simulink subsystem "InversePendulum"  (R2023a)
settings: Solver=VariableStepAuto  StartTime=0.0  StopTime=10.0  RelTol=1e-3
values from neighbouring files (symbols this model uses):
  g = 9.8    [constants.m]
  L = 350 * 10^-6    (= 0.00035)    [constants.m]
  m = .1    (= 0.1)    [constants.m]
  M = .2    (= 0.2)    [constants.m]
  ts = 3/7    (= 0.428571428571)    [constants.m]
settings Model: Creator=ycheb  LastModifiedBy=Edgar

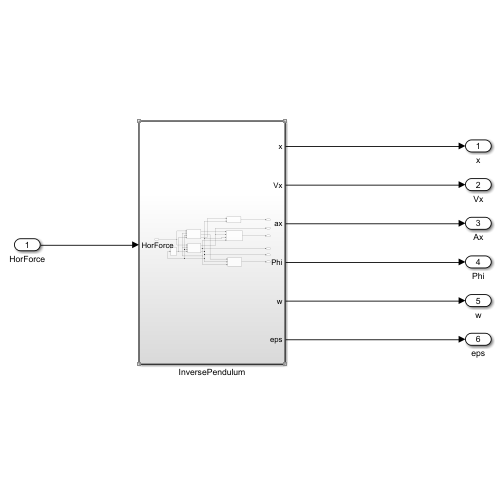
[thumbnail: Simulink's stored preview of the top-level diagram]
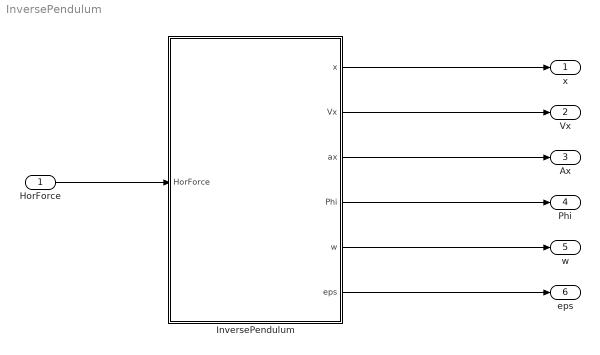
== system InversePendulum ==
  HorForce : Inport
  InversePendulum : Subsystem
  x : Outport
  Vx : Outport  Port=2
  Ax : Outport  Port=3
  Phi : Outport  Port=4
  w : Outport  Port=5
  eps : Outport  Port=6
  wires:
  InversePendulum/5(w) -> w/1
  InversePendulum/4(Phi) -> Phi/1
  InversePendulum/6(eps) -> eps/1
  InversePendulum/2(Vx) -> Vx/1
  HorForce/1 -> InversePendulum/1(HorForce)
  InversePendulum/3(ax) -> Ax/1
  InversePendulum/1(x) -> x/1

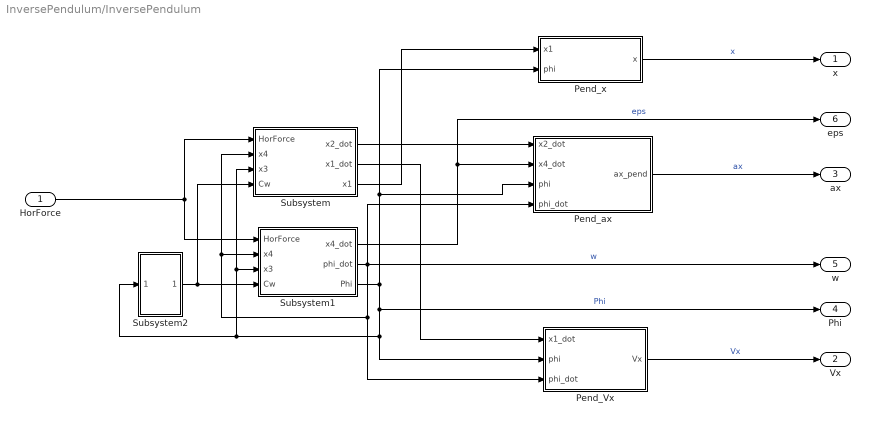
== system InversePendulum/InversePendulum ==
  HorForce : Inport
  Pend_Vx : Subsystem
  Pend_ax : Subsystem
  Pend_x : Subsystem
  Subsystem : Subsystem
  Subsystem1 : Subsystem
  Subsystem2 : Subsystem
  x : Outport
  Vx : Outport  Port=2
  ax : Outport  Port=3
  Phi : Outport  Port=4
  w : Outport  Port=5
  eps : Outport  Port=6
  wires:
  Subsystem1/2(phi_dot) -> w/1, Pend_ax/4(phi_dot), Pend_Vx/3(phi_dot), Subsystem/2(x4), Subsystem1/2(x4)  "w"
  Subsystem2/1(Cw) -> Subsystem/4(Cw), Subsystem1/4(Cw)
  HorForce/1 -> Subsystem1/1(HorForce), Subsystem/1(HorForce)
  Subsystem1/3(Phi) -> Phi/1, Pend_Vx/2(phi), Subsystem/3(x3), Subsystem1/3(x3), Subsystem2/1(Phi), Pend_x/2(phi), Pend_ax/3(phi)  "Phi"
  Pend_Vx/1(Vx) -> Vx/1  "Vx"
  Pend_ax/1(ax_pend) -> ax/1  "ax"
  Subsystem1/1(x4_dot) -> eps/1, Pend_ax/2(x4_dot)  "eps"
  Subsystem/1(x2_dot) -> Pend_ax/1(x2_dot)
  Subsystem/3(x1) -> Pend_x/1(x1)
  Subsystem/2(x1_dot) -> Pend_Vx/1(x1_dot)
  Pend_x/1(x) -> x/1  "x"

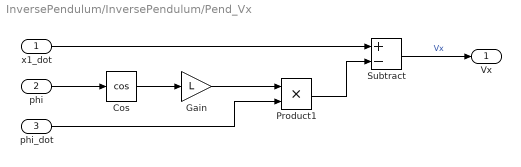
== system InversePendulum/InversePendulum/Pend_Vx ==
  x1_dot : Inport
  phi : Inport  Port=2
  phi_dot : Inport  Port=3
  Cos : Trigonometry  Operator=cos
  Gain : Gain  Gain=L
  Product1 : Product
  Subtract : Sum  Inputs=+-
  Vx : Outport
  wires:
  phi/1 -> Cos/1
  Subtract/1 -> Vx/1  "Vx"
  x1_dot/1 -> Subtract/1
  phi_dot/1 -> Product1/2
  Product1/1 -> Subtract/2
  Cos/1 -> Gain/1
  Gain/1 -> Product1/1

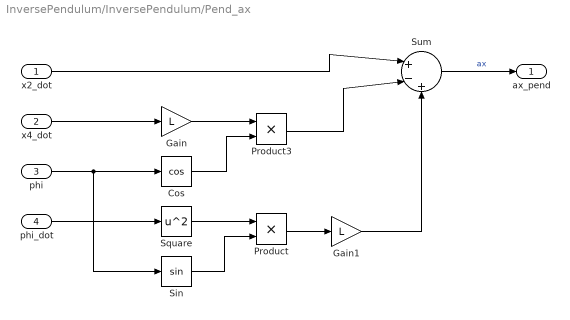
== system InversePendulum/InversePendulum/Pend_ax ==
  x2_dot : Inport
  x4_dot : Inport  Port=2
  phi : Inport  Port=3
  phi_dot : Inport  Port=4
  Cos : Trigonometry  Operator=cos
  Gain : Gain  Gain=L
  Gain1 : Gain  Gain=L
  Product : Product
  Product3 : Product
  Sin : Trigonometry
  Square : Math  Operator=square
  Sum : Sum  Inputs=|+-+
  ax_pend : Outport
  wires:
  x2_dot/1 -> Sum/1
  Sum/1 -> ax_pend/1  "ax"
  Gain/1 -> Product3/1
  Product3/1 -> Sum/2
  phi/1 -> Sin/1, Cos/1
  Cos/1 -> Product3/2
  x4_dot/1 -> Gain/1
  phi_dot/1 -> Square/1
  Square/1 -> Product/1
  Sin/1 -> Product/2
  Product/1 -> Gain1/1
  Gain1/1 -> Sum/3

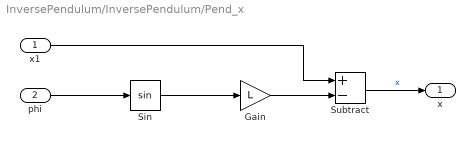
== system InversePendulum/InversePendulum/Pend_x ==
  x1 : Inport
  phi : Inport  Port=2
  Gain : Gain  Gain=L
  Sin : Trigonometry
  Subtract : Sum  Inputs=+-
  x : Outport
  wires:
  Sin/1 -> Gain/1
  Gain/1 -> Subtract/2
  Subtract/1 -> x/1  "x"
  x1/1 -> Subtract/1
  phi/1 -> Sin/1

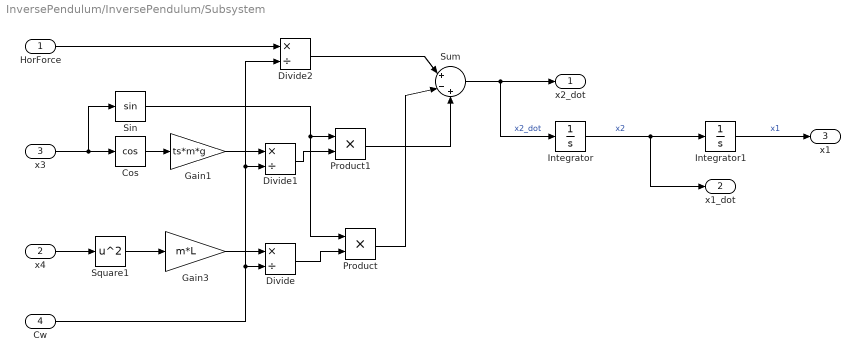
== system InversePendulum/InversePendulum/Subsystem ==
  HorForce : Inport
  x4 : Inport  Port=2
  x3 : Inport  Port=3
  Cw : Inport  Port=4
  Cos : Trigonometry  Operator=cos
  Divide : Product  Inputs=*/
  Divide1 : Product  Inputs=*/
  Divide2 : Product  Inputs=*/
  Gain1 : Gain  Gain=ts*m*g
  Gain3 : Gain  Gain=m*L
  Integrator : Integrator
  Integrator1 : Integrator
  Product : Product
  Product1 : Product
  Sin : Trigonometry
  Square1 : Math  Operator=square
  Sum : Sum  Inputs=|+-+
  x2_dot : Outport
  x1_dot : Outport  Port=2
  x1 : Outport  Port=3
  wires:
  Sum/1 -> Integrator/1, x2_dot/1  "x2_dot"
  Square1/1 -> Gain3/1
  Product/1 -> Sum/2
  x3/1 -> Sin/1, Cos/1
  x4/1 -> Square1/1
  Integrator/1 -> x1_dot/1, Integrator1/1  "x2"
  Integrator1/1 -> x1/1  "x1"
  Cos/1 -> Gain1/1
  Sin/1 -> Product/1, Product1/1
  Product1/1 -> Sum/3
  Gain3/1 -> Divide/1
  Cw/1 -> Divide/2, Divide2/2, Divide1/2
  Divide/1 -> Product/2
  Gain1/1 -> Divide1/1
  Divide1/1 -> Product1/2
  HorForce/1 -> Divide2/1
  Divide2/1 -> Sum/1

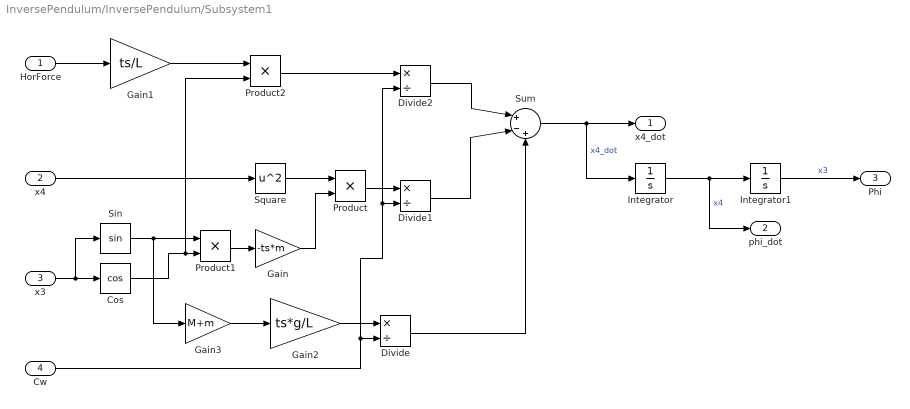
== system InversePendulum/InversePendulum/Subsystem1 ==
  HorForce : Inport
  x4 : Inport  Port=2
  x3 : Inport  Port=3
  Cw : Inport  Port=4
  Cos : Trigonometry  Operator=cos
  Divide : Product  Inputs=*/
  Divide1 : Product  Inputs=*/
  Divide2 : Product  Inputs=*/
  Gain : Gain  Gain=-ts*m
  Gain1 : Gain  Gain=ts/L
  Gain2 : Gain  Gain=ts*g/L
  Gain3 : Gain  Gain=M+m
  Integrator : Integrator
  Integrator1 : Integrator  InitialCondition=5*pi/180
  Product : Product
  Product1 : Product
  Product2 : Product
  Sin : Trigonometry
  Square : Math  Operator=square
  Sum : Sum  Inputs=|+-+
  x4_dot : Outport
  phi_dot : Outport  Port=2
  Phi : Outport  Port=3
  wires:
  Gain/1 -> Product/2
  x3/1 -> Cos/1, Sin/1
  Square/1 -> Product/1
  Gain3/1 -> Gain2/1
  Sum/1 -> Integrator/1, x4_dot/1  "x4_dot"
  HorForce/1 -> Gain1/1
  x4/1 -> Square/1
  Integrator/1 -> Integrator1/1, phi_dot/1  "x4"
  Integrator1/1 -> Phi/1  "x3"
  Sin/1 -> Gain3/1, Product1/1
  Cos/1 -> Product1/2, Product2/2
  Product1/1 -> Gain/1
  Gain1/1 -> Product2/1
  Gain2/1 -> Divide/1
  Cw/1 -> Divide/2, Divide2/2, Divide1/2
  Divide/1 -> Sum/3
  Product/1 -> Divide1/1
  Divide1/1 -> Sum/2
  Product2/1 -> Divide2/1
  Divide2/1 -> Sum/1

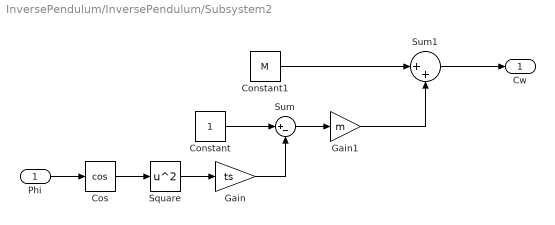
== system InversePendulum/InversePendulum/Subsystem2 ==
  Phi : Inport
  Constant : Constant
  Constant1 : Constant  Value=M
  Cos : Trigonometry  Operator=cos
  Gain : Gain  Gain=ts
  Gain1 : Gain  Gain=m
  Square : Math  Operator=square
  Sum : Sum  Inputs=|+-
  Sum1 : Sum  Inputs=|++
  Cw : Outport
  wires:
  Phi/1 -> Cos/1
  Cos/1 -> Square/1
  Square/1 -> Gain/1
  Gain/1 -> Sum/2
  Constant/1 -> Sum/1
  Sum/1 -> Gain1/1
  Constant1/1 -> Sum1/1
  Gain1/1 -> Sum1/2
  Sum1/1 -> Cw/1
